simulink model "computedtroqwithgaitsim"  (R2019a)
settings: Solver=ode23  StartTime=0.0  StopTime=10  MaxStep=0.02  RelTol=1e-3
settings Model: Creator=zkibria  LastModifiedBy=zkibria

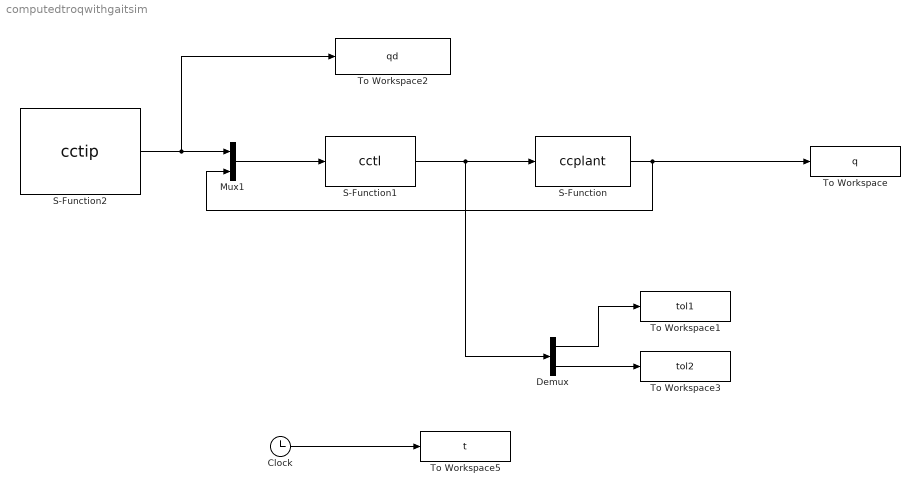
== system computedtroqwithgaitsim ==
  Clock : Clock
  Demux : Demux  Outputs=2
  Mux1 : Mux  Inputs=2
  S-Function : S-Function  FunctionName=ccplant  SFunctionDeploymentMode=off  EnableBusSupport=off
  S-Function1 : S-Function  FunctionName=cctl  SFunctionDeploymentMode=off  EnableBusSupport=off
  S-Function2 : S-Function  FunctionName=cctip  SFunctionDeploymentMode=off  EnableBusSupport=off
  To Workspace : ToWorkspace  VariableName=q  SaveFormat=Timeseries  SampleTime=-1
  To Workspace1 : ToWorkspace  VariableName=tol1  SaveFormat=Timeseries  SampleTime=-1
  To Workspace2 : ToWorkspace  VariableName=qd  SaveFormat=Timeseries  SampleTime=-1
  To Workspace3 : ToWorkspace  VariableName=tol2  SaveFormat=Timeseries  SampleTime=-1
  To Workspace5 : ToWorkspace  VariableName=t  SaveFormat=Timeseries  SampleTime=-1
  wires:
  Clock/1 -> To Workspace5/1
  S-Function2/1 -> To Workspace2/1, Mux1/1
  Mux1/1 -> S-Function1/1
  S-Function1/1 -> Demux/1, S-Function/1
  S-Function/1 -> To Workspace/1, Mux1/2
  Demux/1 -> To Workspace1/1
  Demux/2 -> To Workspace3/1
